simulink model "ex22"  (R2021a)
settings: Solver=VariableStepAuto  StartTime=0.0  StopTime=10.0  RelTol=1e-3
undefined symbols (not defined in the file or in its folder): g, k, kd, m, omegas
settings Model: Creator=frede  LastModifiedBy=frede

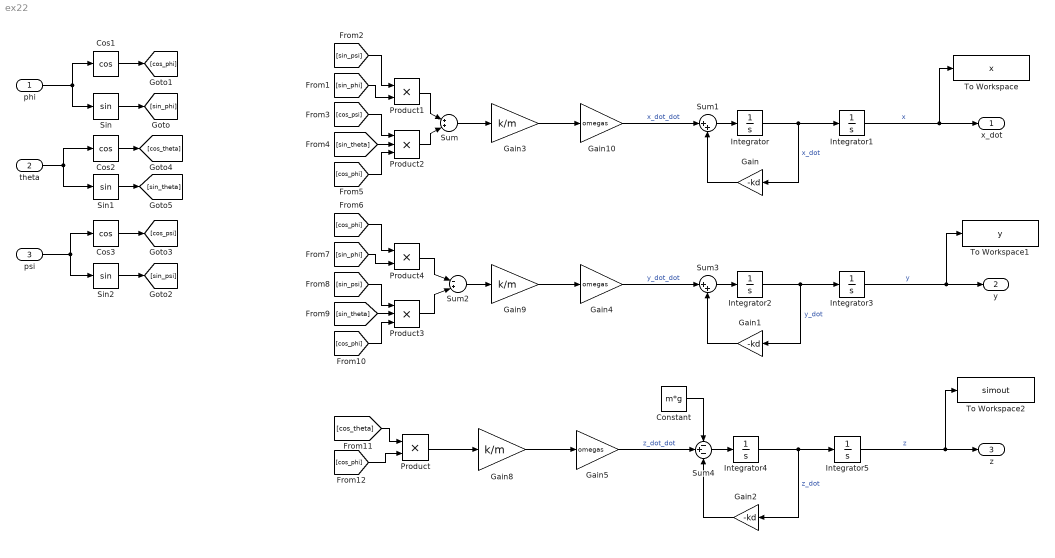
== system ex22 ==
  phi : Inport
  theta : Inport  Port=2
  psi : Inport  Port=3
  Constant : Constant  Value=m*g
  Cos1 : Trigonometry  Operator=cos
  Cos2 : Trigonometry  Operator=cos
  Cos3 : Trigonometry  Operator=cos
  Gain : Gain  Gain=-kd
  Gain1 : Gain  Gain=-kd
  Gain10 : Gain  Gain=omegas
  Gain2 : Gain  Gain=-kd
  Gain3 : Gain  Gain=k/m
  Gain4 : Gain  Gain=omegas
  Gain5 : Gain  Gain=omegas
  Gain8 : Gain  Gain=k/m
  Gain9 : Gain  Gain=k/m
  Integrator{,1..5} (6 alike) : Integrator
  Product : Product
  Product1 : Product
  Product2 : Product  Inputs=3
  Product3 : Product  Inputs=3
  Product4 : Product
  Sin : Trigonometry
  Sin1 : Trigonometry
  Sin2 : Trigonometry
  Sum : Sum  Inputs=|++|
  Sum1 : Sum  Inputs=|++
  Sum2 : Sum  Inputs=|-+|
  Sum3 : Sum  Inputs=|++
  Sum4 : Sum  Inputs=-+-
  To Workspace : ToWorkspace  VariableName=x  SaveFormat=Timeseries  SampleTime=-1
  To Workspace1 : ToWorkspace  VariableName=y  SaveFormat=Timeseries  SampleTime=-1
  To Workspace2 : ToWorkspace  VariableName=simout  SaveFormat=Timeseries  SampleTime=-1
  x_dot : Outport
  y : Outport  Port=2
  z : Outport  Port=3
  wires:
  [cos_phi] -> Product4/1
  Gain1/1 -> Sum3/2
  Cos1/1 -> [cos_phi]
  Sin/1 -> [sin_phi]
  Gain8/1 -> Gain5/1
  Product/1 -> Gain8/1
  Integrator5/1 -> To Workspace2/1, z/1  "z"
  Integrator2/1 -> Gain1/1, Integrator3/1  "y_dot"
  Product4/1 -> Sum2/1
  Gain2/1 -> Sum4/3
  theta/1 -> Sin1/1, Cos2/1
  [sin_theta] -> Product3/2
  [cos_phi] -> Product/2
  [cos_psi] -> Product2/1
  [sin_psi] -> Product1/1
  Constant/1 -> Sum4/1
  Sin2/1 -> [sin_psi]
  Integrator/1 -> Gain/1, Integrator1/1  "x_dot"
  Sin1/1 -> [sin_theta]
  Integrator3/1 -> y/1, To Workspace1/1  "y"
  psi/1 -> Sin2/1, Cos3/1
  Sum4/1 -> Integrator4/1
  Sum2/1 -> Gain9/1
  Gain9/1 -> Gain4/1
  Sum1/1 -> Integrator/1
  Gain/1 -> Sum1/2
  Product2/1 -> Sum/2
  Gain3/1 -> Gain10/1
  Gain4/1 -> Sum3/1  "y_dot_dot"
  [sin_phi] -> Product1/2
  Sum3/1 -> Integrator2/1
  Cos3/1 -> [cos_psi]
  [cos_theta] -> Product/1
  [sin_phi] -> Product4/2
  Integrator1/1 -> To Workspace/1, x_dot/1  "x"
  phi/1 -> Cos1/1, Sin/1
  Gain10/1 -> Sum1/1  "x_dot_dot"
  Product1/1 -> Sum/1
  [cos_phi] -> Product3/3
  Integrator4/1 -> Gain2/1, Integrator5/1  "z_dot"
  Gain5/1 -> Sum4/2  "z_dot_dot"
  [sin_theta] -> Product2/2
  [cos_phi] -> Product2/3
  Cos2/1 -> [cos_theta]
  [sin_psi] -> Product3/1
  Product3/1 -> Sum2/2
  Sum/1 -> Gain3/1
